simulink model "Observador_Nuevo"  (R2013b)
settings: Solver=ode45  StartTime=0.0  StopTime=10  MaxStep=0.01  RelTol=1e-3
values from neighbouring files (symbols this model uses):
  A = [0 1; -Mt/I -Kf/I]    [HinfPlantSeguroa.m]    (also in HinfPlanta.m)
  B = [0; L1/I]    [HinfPlantSeguroa.m]    (also in HinfPlanta.m)
  C = [1 0]    [HinfPlantSeguroa.m]    (also in HinfPlanta.m)
  L = G1*K1    [HinfPlantSeguroa.m]    (also in HinfPlanta.m)
settings Model: CovModelRefEnable=off  Creator=i95sa  LastModifiedBy=Mecatronica
settings DataIOCC: LimitDataPoints=off  SaveFormat=StructureWithTime
settings DebuggingCC: UnderspecifiedInitializationDetection=Simplified  MergeDetectMultiDrivingBlocksExec=error  SolverPrmCheckMsg=none  FcnCallInpInsideContextMsg=EnableAllAsWarning  FrameProcessingCompatibilityMsg=error
settings HardwareCC: ProdBitPerPointer=64  ProdLargestAtomicFloat=Float  ProdIntDivRoundTo=Zero  ProdEndianess=LittleEndian  ProdHWDeviceType=Specified
settings ModelReferenceCC: PropagateSignalLabelsOutOfModel=on
settings GRTTargetCC: CodeReplacementLibrary=C89/C90 (ANSI)

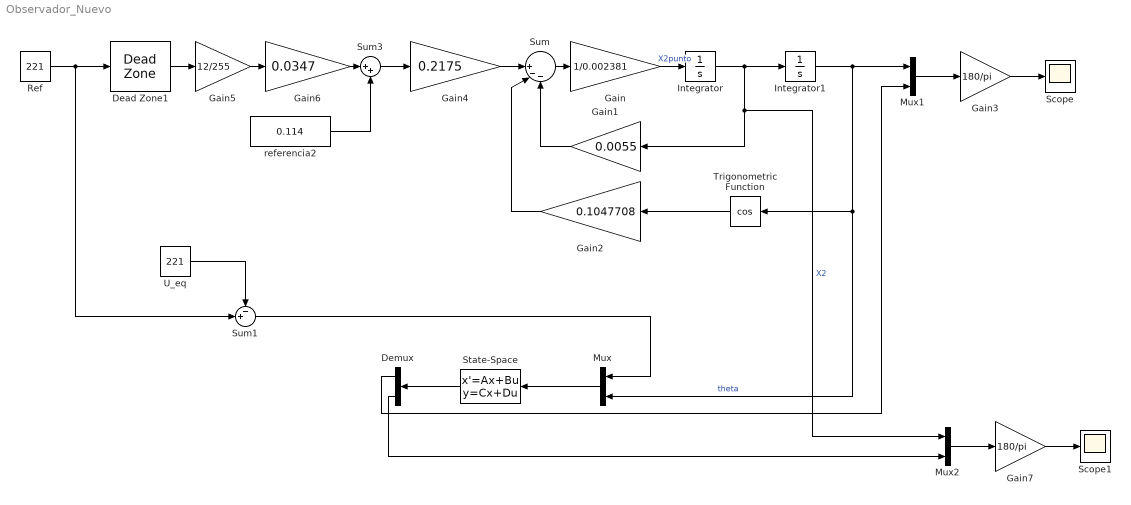
== system Observador_Nuevo ==
  Dead Zone1 : DeadZone  LowerValue=0  UpperValue=0  SaturateOnIntegerOverflow=on
  Demux : Demux  Outputs=2
  Gain : Gain  Gain=1/0.002381
  Gain1 : Gain  Gain=0.0055
  Gain2 : Gain  Gain=0.1047708
  Gain3 : Gain  Gain=180/pi
  Gain4 : Gain  Gain=0.2175
  Gain5 : Gain  Gain=12/255
  Gain6 : Gain  Gain=0.0347
  Gain7 : Gain  Gain=180/pi
  Integrator : Integrator
  Integrator1 : Integrator  InitialCondition=-0.65
  Mux : Mux  Inputs=2
  Mux1 : Mux  Inputs=2
  Mux2 : Mux  Inputs=2
  Ref : Constant  Value=221
  Scope : Scope
  Scope1 : Scope
  State-Space : StateSpace  A=A-L*C  B=[B L]  C=eye(2)  D=zeros(2,2)  X0=[-0.65 0]
  Sum : Sum  Inputs=||+--
  Sum1 : Sum  Inputs=-+|
  Sum3 : Sum  Inputs=|++
  Trigonometric Function : Trigonometry  Operator=cos
  U_eq : Constant  Value=221
  referencia2 : Constant  Value=0.114
  wires:
  Sum/1 -> Gain/1
  Gain/1 -> Integrator/1  "X2punto"
  Integrator/1 -> Integrator1/1, Mux2/1, Gain1/1  "X2"
  Trigonometric Function/1 -> Gain2/1
  Gain1/1 -> Sum/3
  Integrator1/1 -> Mux1/1, Mux/2, Trigonometric Function/1  "theta"
  Gain2/1 -> Sum/2
  Gain4/1 -> Sum/1
  referencia2/1 -> Sum3/2
  Sum3/1 -> Gain4/1
  Gain5/1 -> Gain6/1
  Gain6/1 -> Sum3/1
  Dead Zone1/1 -> Gain5/1
  Gain3/1 -> Scope/1
  State-Space/1 -> Demux/1
  Mux/1 -> State-Space/1
  Ref/1 -> Sum1/2, Dead Zone1/1
  Sum1/1 -> Mux/1
  U_eq/1 -> Sum1/1
  Mux1/1 -> Gain3/1
  Gain7/1 -> Scope1/1
  Mux2/1 -> Gain7/1
  Demux/1 -> Mux1/2
  Demux/2 -> Mux2/2
